simulink model "Factorial_Task"  (R2021a)
settings: Solver=FixedStepDiscrete  StartTime=0.0  StopTime=10.0  RelTol=1e-3  EnableMultiTasking=on
settings Model: Creator=elkny  LastModifiedBy=elkny
settings DataIOCC: ReturnWorkspaceOutputs=off
settings OptimizationCC: DefaultParameterBehavior=Inlined  InlineInvariantSignals=on  EnableMemcpy=off  LifeSpan=1  EfficientTunableParamExpr=on
settings DebuggingCC: UnderspecifiedInitializationDetection=Classic  MergeDetectMultiDrivingBlocksExec=none  SFMachineParentedDataDiag=warning  ArithmeticOperatorsInVariantConditions=warning
settings ModelReferenceCC: PropagateSignalLabelsOutOfModel=off
settings SFSimCC: MATLABDynamicMemAlloc=off  CustomCodeUndefinedFunction=UseInterfaceOnly
settings RTWCC: SystemTargetFile=ert.tlc  GenCodeOnly=on  TemplateMakefile=ert_default_tmf  GenerateReport=on  IncludeHyperlinkInReport=on  LaunchReport=on  GenerateTraceInfo=on  GenerateTraceReport=on  GenerateTraceReportSl=on  GenerateTraceReportSf=on  GenerateTraceReportEml=on
settings CodeAppCC: ForceParamTrailComments=on  IgnoreCustomStorageClasses=off  OperatorAnnotations=on  SimulinkDataObjDesc=on  SFDataObjDesc=on  MATLABFcnDesc=on  InsertBlockDesc=on  StateflowObjectComments=on  MATLABSourceComments=on
settings ERTTargetCC: MultiwordLength=2048  GenerateSampleERTMain=on  InlinedParameterPlacement=NonHierarchical  ERTCustomFileTemplate=example_file_process.tlc

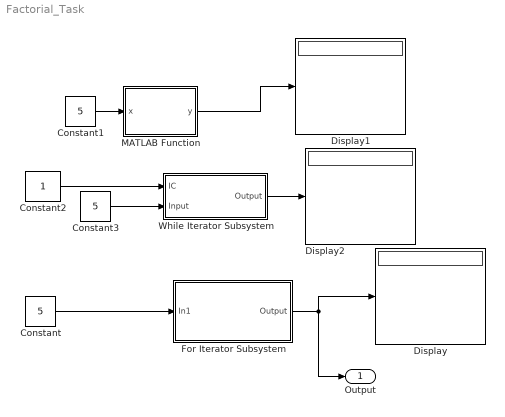
== system Factorial_Task ==
  Constant : Constant  Value=5  OutDataTypeStr=uint32
  Constant1 : Constant  Value=5  OutDataTypeStr=uint32
  Constant2 : Constant
  Constant3 : Constant  Value=5  OutDataTypeStr=uint32
  Display : Display
  Display1 : Display
  Display2 : Display
  For Iterator Subsystem : Subsystem  TreatAsAtomicUnit=on
  MATLAB Function : MATLAB Function  TreatAsAtomicUnit=on
  While Iterator Subsystem : Subsystem  TreatAsAtomicUnit=on
  Output : Outport
  wires:
  Constant/1 -> For Iterator Subsystem/1(In1)
  For Iterator Subsystem/1(Output) -> Output/1, Display/1
  Constant1/1 -> MATLAB Function/1(x)
  MATLAB Function/1(y) -> Display1/1
  Constant2/1 -> While Iterator Subsystem/1(IC)
  While Iterator Subsystem/1(Output) -> Display2/1
  Constant3/1 -> While Iterator Subsystem/2(Input)

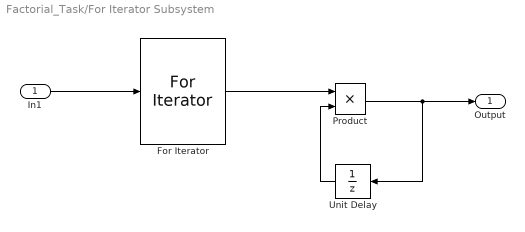
== system Factorial_Task/For Iterator Subsystem ==
  In1 : Inport  OutDataTypeStr=uint32
  For Iterator : ForIterator  IterationSource=external  IterationVariableDataType=uint32
  Product : Product  OutDataTypeStr=uint32
  Unit Delay : UnitDelay  InitialCondition=1  SampleTime=-1  HasFrameUpgradeWarning=on
  Output : Outport
  wires:
  For Iterator/1 -> Product/1
  Product/1 -> Unit Delay/1, Output/1
  In1/1 -> For Iterator/1
  Unit Delay/1 -> Product/2

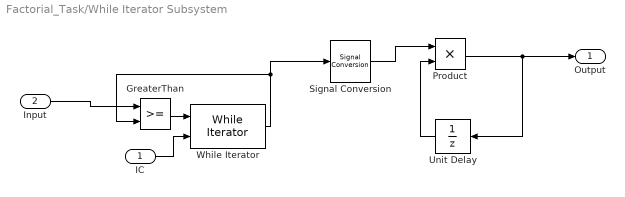
== system Factorial_Task/While Iterator Subsystem ==
  IC : Inport
  Input : Inport  Port=2
  GreaterThan : RelationalOperator  OutDataTypeStr=boolean  RndMeth=Simplest
  Product : Product  OutDataTypeStr=uint32
  Signal Conversion : SignalConversion  OverrideOpt=off
  Unit Delay : UnitDelay  InitialCondition=1  SampleTime=-1  HasFrameUpgradeWarning=on
  While Iterator : WhileIterator  ShowIterationPort=on
  Output : Outport
  wires:
  IC/1 -> While Iterator/2
  Unit Delay/1 -> Product/2
  Product/1 -> Unit Delay/1, Output/1
  GreaterThan/1 -> While Iterator/1
  Input/1 -> GreaterThan/1
  While Iterator/1 -> GreaterThan/2, Signal Conversion/1
  Signal Conversion/1 -> Product/1

== matlab function Factorial_Task/MATLAB Function ==
  data: x input; y output
function y = calculateFactorial(x)
   y=factorial(x);
end
